simulink model "test_UDPreciever_in_simulink"  (R2021b)
settings: Solver=VariableStepAuto  StartTime=0.0  StopTime=1  RelTol=1e-3
libraries: slrealtimeutilitieslib x1, slrealtimeiplib x1
settings Model: Creator=willy  LastModifiedBy=willy

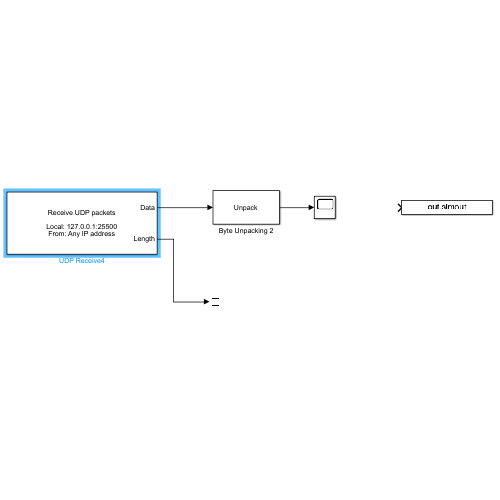
[thumbnail: Simulink's stored preview of the top-level diagram]
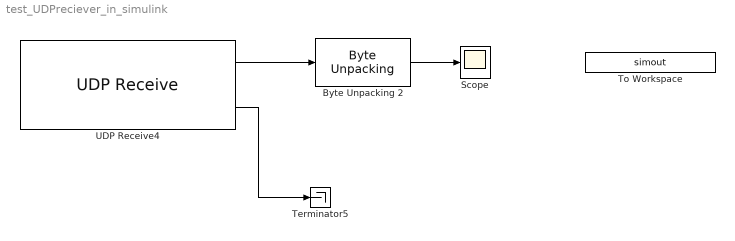
== system test_UDPreciever_in_simulink ==
  Byte Unpacking 2 : slrealtimeutilitieslib/Byte Unpacking  MaskUnpackedDataTypes={'double'}  MaskUnpackedDataSizes={[1]}  MaskAlignment=1
      settings: SourceProductBaseCode=XP
  Scope : Scope
  Terminator5 : Terminator
  To Workspace : ToWorkspace  VariableName=simout  SaveFormat=Timeseries  SampleTime=-1
      settings: MaxDataPoints=1  Decimation=2
  UDP Receive4 : slrealtimeiplib/UDP Receive  useHostTargetConn=off  ipAddress=127.0.0.1  localPort=25500  rcvWidth=8  rcvFmAny=on  fmAddress=127.0.0.0  sampleTime=0.01
      settings: SourceProductBaseCode=XP
  wires:
  UDP Receive4/1 -> Byte Unpacking 2/1
  UDP Receive4/2 -> Terminator5/1
  Byte Unpacking 2/1 -> Scope/1
